simulink model "error_recta"  (R2025b)
settings: Solver=VariableStepAuto  StartTime=0.0  StopTime=inf  RelTol=1e-3
undefined symbols (not defined in the file): gray, Rec, SDTV
libraries: visionconversions x1, dspvision x1
settings Model: Creator=Albert  LastModifiedBy=Albert
settings DataIOCC: ReturnWorkspaceOutputs=off

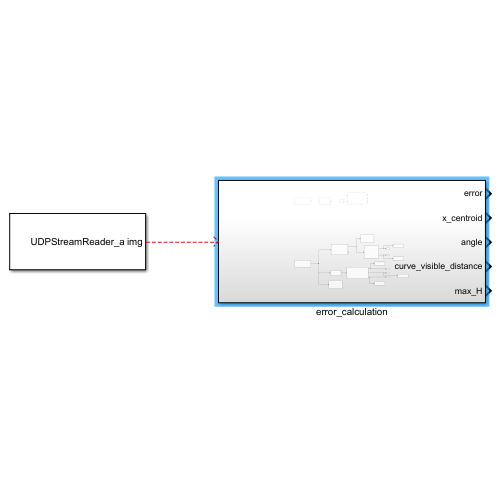
[thumbnail: Simulink's stored preview of the top-level diagram]
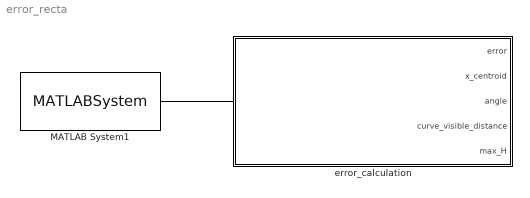
== system error_recta ==
  MATLAB System1 : MATLABSystem  System=UDPStreamReader_a  LocalPort=8888  SimulateUsing=Interpreted execution
      mask Type: UDPStreamReader_a
  error_calculation : Subsystem
  wires:
  MATLAB System1/1 -> ?

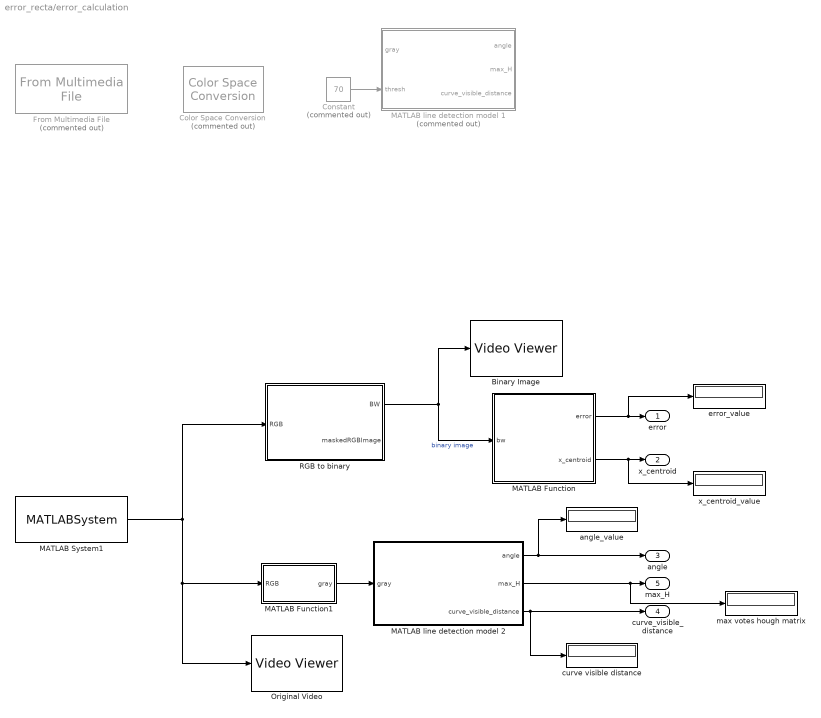
== system error_recta/error_calculation ==
  Binary Image : VideoViewer  colormapValue=gray(256)  FigPos=[240 625 418 304]
  Color Space Conversion : visionconversions/Color Space  Conversion  Commented=on  conversion=Obsolete  conversionActive=R'G'B' to intensity  wp_str=D65  rec=Rec. 601 (SDTV)  sys=1125/60/2:1  imagePorts=One multidimensional signal
  Constant : Constant  Commented=on  Value=70
  From Multimedia File : dspvision/From Multimedia File  Commented=on  inputFilename=C:\Users\Albert\Desktop\AAUNI\AATFG\Videos_cinta\Recta_cinta.mp4  readRange=[1 Inf]  loop=on  numPlays=inf  outputStreams=Video only  videoDataType=uint8  audioDataType=int16  inheritSampleTime=on  userDefinedSampleTime=1/30  noAudioOutput=off  isIntensityVideo=off  fourcc=RGB  colorVideoFormat=One multidimensional signal  outputEOF=off  dataOrg=Column-major  audioFrameSize=1024  computeAudioFrameSize=off  outSamplingMode=Sample based
      settings: LibrarySourceBlock=visionsources/From Multimedia File
  MATLAB Function : MATLAB Function  TreatAsAtomicUnit=on
  MATLAB Function1 : MATLAB Function  TreatAsAtomicUnit=on
  MATLAB System1 : MATLABSystem  System=UDPStreamReader_a  LocalPort=8888  SimulateUsing=Interpreted execution
      mask Type: UDPStreamReader_a
  MATLAB line detection model 1 : MATLAB Function  Commented=on  TreatAsAtomicUnit=on
  MATLAB line detection model 2 : MATLAB Function  TreatAsAtomicUnit=on
  Original Video : VideoViewer  colormapValue=gray(256)  FigPos=[660 620 418 304]
  RGB to binary : MATLAB Function  TreatAsAtomicUnit=on
  angle_value : Display
  curve visible distance : Display
  error_value : Display
  max votes hough matrix : Display
  x_centroid_value : Display
  error : Outport
  x_centroid : Outport  Port=2
  angle : Outport  Port=3
  curve_visible_distance : Outport  Port=4
  max_H : Outport  Port=5
  wires:
  MATLAB Function/2(x_centroid) -> x_centroid/1, x_centroid_value/1
  MATLAB Function/1(error) -> error_value/1, error/1
  RGB to binary/1(BW) -> Binary Image/1, MATLAB Function/1(bw)  "binary image"
  MATLAB System1/1 -> RGB to binary/1(RGB), Original Video/1, MATLAB Function1/1(RGB)
  MATLAB Function1/1(gray) -> MATLAB line detection model 2/1(gray)
  MATLAB line detection model 2/1(angle) -> angle_value/1, angle/1
  MATLAB line detection model 2/3(curve_visible_distance) -> curve_visible_distance/1, curve visible distance/1
  Constant/1 -> MATLAB line detection model 1/2(thresh)
  MATLAB line detection model 2/2(max_H) -> max votes hough matrix/1, max_H/1

== matlab function error_recta/error_calculation/RGB to binary ==
  data: BW output; RGB input; maskedRGBImage output
function [BW,maskedRGBImage] = createMask(RGB)
%createMask  Threshold RGB image using auto-generated code from colorThresholder app.
%  [BW,MASKEDRGBIMAGE] = createMask(RGB) thresholds image RGB using
%  auto-generated code from the colorThresholder app. The colorspace and
%  range for each channel of the colorspace were set within the app. The
%  segmentation mask is returned in BW, and a composite of the mask and
%  original RGB images is returned in maskedRGBImage.

% Auto-generated by colorThresholder app on 12-Sep-2026
%------------------------------------------------------


% Convert RGB image to chosen color space
I = rgb2hsv(RGB);

% Define thresholds for channel 1 based on histogram settings
channel1Min = 0.984;
channel1Max = 0.142;

% Define thresholds for channel 2 based on histogram settings
channel2Min = 0.244;
channel2Max = 1.000;

% Define thresholds for channel 3 based on histogram settings
channel3Min = 0.000;
channel3Max = 1.000;

% Create mask based on chosen histogram thresholds
sliderBW = ( (I(:,:,1) >= channel1Min) | (I(:,:,1) <= channel1Max) ) & ...
    (I(:,:,2) >= channel2Min ) & (I(:,:,2) <= channel2Max) & ...
    (I(:,:,3) >= channel3Min ) & (I(:,:,3) <= channel3Max);
BW = sliderBW;
% BW = bwareaopen(BW2, 100);

% Initialize output masked image based on input image.
maskedRGBImage = RGB;

% Set background pixels where BW is false to zero.
maskedRGBImage(repmat(~BW,[1 1 3])) = 0;

end

% function bw = otsu_binarize(img)
% 
% norm = graythresh(img);
% bw = imbinarize(img, norm);
% 
% end

% function bw = otsu_binarize(img)
%     % Calculate average image brightness and apply offset
%     thresh = mean(img(:) - 0.05); % Adjust offset between 0.1 and 0.3 if needed
% 
%     % Return binary matrix directly
%     bw = img > thresh;
% end

== matlab function error_recta/error_calculation/MATLAB Function ==
  data: bw input; error output; x_centroid output
function [error, x_centroid] = calculate_line_error(bw)
    % Image resolution from Video Viewer: 480 rows x 640 columns
    [height, width] = size(bw);
    x_center = width / 2; % Image center is x = 320

    % Focus on a Region of Interest (ROI) at the bottom 25% of the frame
    roi_start = round(height * 0.75);
    roi = bw(roi_start:end, :); % bw(files, columnes) == bw(from roi_start to end (Yaxis), from begining to end (Xaxis)

    % Find column coordinates where line pixels (1s) exist
    [~, cols] = find(roi > 0);
    % cols = [1; 2; 2] (exemple diferent)
    
    if ~isempty(cols) % = if 1 then
        x_centroid = mean(cols);     % Calculate average X-position of line
        error = x_centroid - x_center; % Lateral distance from center
    else % = else (if 0 then)
        x_centroid = x_center;        % Fallback if line is lost
        error = 0;
    end
end


% function[error, x_centroid, v] = error_and_velocityControl(bw)
% 
% [height, width] = size(bw); % 480 x 640
% x_center = width / 2; % Image center is x = 320
% 
% % Focus on the two Regions of Interest (lower for error calculation and 
% roi_start = round(height * 0.5);
% 
% roi2 = bw(1:roi_start - 1,:); % Des de l'altura fins a la meitat (50% superior)
% roi1 = bw(roi_start:end, :); % bw(rows, cols) == bw(from roi_start to end (Yaxis), from begining to end (Xaxis) ----> Top row == 1, bottom row == height!
% 
% % LOWER ROI (ROI1)
% [num_rows_roi1, num_cols_roi1] = size(roi1);
% suma_posiciones = 0;
% suma_unos = 0;
% 
% for col = 1:num_cols_roi1
%     for row = 1:num_rows_roi1
%         if roi1(row, col) == 1
%             suma_posiciones = suma_posiciones + col; % Follows centroid formula sum(position_x) / number of ones
%             suma_unos = suma_unos + 1; % Follows centroid formula sum(position_x) / number of ones
%         end
%     end
% end
% if suma_unos > 0 
%     x_centroid = suma_posiciones / suma_unos;
% else
%     x_centroid = num_cols_roi1 / 2;
% end
% error = x_center - x_centroid;
% 
% % UPPER ROI (ROI2) Track anticipation
% end

== matlab function error_recta/error_calculation/MATLAB Function1 ==
  data: RGB input; gray output
function gray = fcn(RGB)

gray = im2gray(RGB);

end

== matlab function error_recta/error_calculation/MATLAB line detection model 1 ==
  data: gray input; angle output; max_H output; curve_visible_distance output; thresh input
function [angle, max_H, curve_visible_distance] = hough_line_detection(gray, thresh)

prewittImg = edge(gray, 'prewitt');             % Canny (filtratge pre)

% GRAY IMAGE EDGE CUT
prewittImg(1:20,:) = 0; % fila, columna
prewittImg(:,1:40) = 0;
prewittImg(:,300:320) = 0;
prewittImg(230:240,:) = 0;

[H, T, R] = hough(prewittImg);                  % H emmagatzema el compte de vots de la im binària de vores. 
max_H = max(H,[],"all");

P = houghpeaks(H, 10, 'Threshold', thresh);     % Matriu conté coordenades 
                                                % dels peaks, no el valor d'aquests                                          
if 	isempty(P)
    angle = 0;
    curve_visible_distance = 0;
    disp("0 lines detected");    
else
    lines_hough = houghlines(prewittImg, T, R, P,"FillGap",5,"MinLength",50); % lines_hough = houghlines(img, theta, rho, peaks, línies amb distància 
    angle = lines_hough(1).theta;
    curve_visible_distance = lines_hough(1).point1(1,2);
end                                          
end

== matlab function error_recta/error_calculation/MATLAB line detection model 2 ==
  data: gray input; angle output; max_H output; curve_visible_distance output
function [angle, max_H, curve_visible_distance] = hough_line_detection(gray)

prewittImg = edge(gray, 'prewitt');             % Canny (filtratge pre)

% GRAY IMAGE EDGE CUT
prewittImg(1:10,:) = 0; % fila, columna
prewittImg(:,1:10) = 0;
prewittImg(:,end - 10:end) = 0;
prewittImg(end - 10:end,:) = 0;

[H, T, R] = hough(prewittImg);                  % H emmagatzema el compte de vots de la im binària de vores. 
max_H = max(H,[],"all");

thresh = max_H;
P = houghpeaks(H, 10, 'Threshold', thresh);     % Matriu conté coordenades
                                                % dels peaks, no el valor d'aquests
lines_hough = houghlines(prewittImg, T, R, P,"FillGap",5,"MinLength",50); % lines_hough = houghlines(img, theta, rho, peaks, línies amb distància
if isempty(lines_hough)
    angle = 0;
    curve_visible_distance = 0;
    disp('no lines detected');
else
    angle = lines_hough(1).theta;
    curve_visible_distance = lines_hough(1).point1(1,2); % !!!! dist visible camera i cal revisar resultat
    disp(['angle = ', num2str(angle)]);
    disp(['distance = ', num2str(curve_visible_distance)]);
end
end
